simulink model "p1g4"  (R2018a)
settings: Solver=VariableStepAuto  StartTime=0.0  StopTime=10  MaxStep=1e-3  RelTol=1e-3
values from neighbouring files (symbols this model uses):
  K1 = 10    [ef.m]
  K2 = 3    [ef.m]
  Ka = 1    [ef.m]
  Ks = 1.5    [ef.m]
  L = 0.2    [ef.m]
  R = 0.1    [ef.m]
  ta = 0.4    [ef.m]
settings Model: Creator=carma  LastModifiedBy=carma

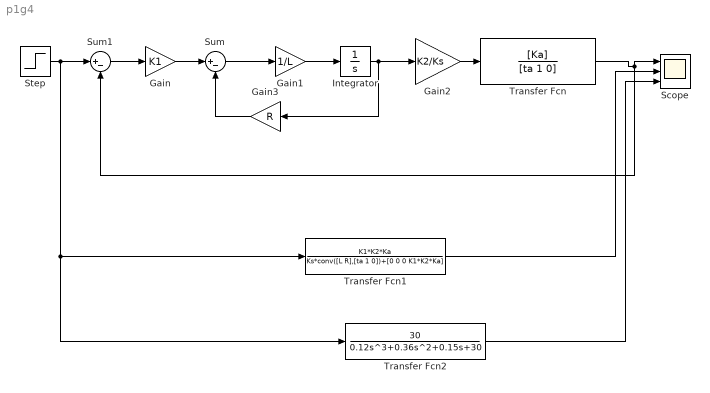
== system p1g4 ==
  Gain : Gain  Gain=K1
  Gain1 : Gain  Gain=1/L
  Gain2 : Gain  Gain=K2/Ks
  Gain3 : Gain  Gain=R
  Integrator : Integrator
  Scope : Scope  NumInputPorts=3
  Step : Step  Time=0  SampleTime=0
  Sum : Sum  Inputs=|+-
  Sum1 : Sum  Inputs=|+-
  Transfer Fcn : TransferFcn  Numerator=[Ka]  Denominator=[ta 1 0]
  Transfer Fcn1 : TransferFcn  Numerator=K1*K2*Ka  Denominator=Ks*conv([L R],[ta 1 0])+[0 0 0 K1*K2*Ka]
  Transfer Fcn2 : TransferFcn  Numerator=30  Denominator=[0.12 0.36 0.15 30]
  wires:
  Gain/1 -> Sum/1
  Sum/1 -> Gain1/1
  Gain1/1 -> Integrator/1
  Integrator/1 -> Gain3/1, Gain2/1
  Gain2/1 -> Transfer Fcn/1
  Transfer Fcn/1 -> Sum1/2, Scope/1
  Gain3/1 -> Sum/2
  Sum1/1 -> Gain/1
  Step/1 -> Transfer Fcn2/1, Transfer Fcn1/1, Sum1/1
  Transfer Fcn1/1 -> Scope/2
  Transfer Fcn2/1 -> Scope/3
